simulink library "Saturation_Value_Water"  (Simulink 8.2)
settings: Solver=ode45  StartTime=0.0  StopTime=10.0  RelTol=1e-3
undefined symbols (not defined in the file): CarnotCallbacks_Saturation_Value_Water
settings Model: Creator=lena.frank  LastModifiedBy=drhf

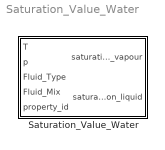
== system Saturation_Value_Water ==
  Saturation_Value_Water : Subsystem  LoadFcn=CarnotCallbacks_Saturation_Value_Water('LoadFcn');  InitFcn=load('THB.mat');  VariantControl=CarlibClassic  mask(saturation value water){INPUTARGUMENTS=state variables (classic), DEBUGLEVEL=WARNINGLEVEL, MAXTOTALMESSAGES=inf, MAXCONSECUTIVEMESSAGES=inf, WRITETOFILE=0, FILENAME='errors.txt'}
      mask prompts: INPUTARGUMENTS "Input arguments"; DEBUGLEVEL "Debug level"; MAXTOTALMESSAGES "maximum number of total warning"; MAXCONSECUTIVEMESSAGES "maximum number of consecutive warnings"; WRITETOFILE "write messages to file"; FILENAME "filename for error messages"
      mask help:
      | Calculates the saturation value of fluid by the value of a specified property.
      | Temperature may be a scalar or vector, all other inputs must be scalar.
      | property-ID        property                       unit
      | 1                       density                         [kg/m³]
      | 2                       heat capacity               [J/kgK]
      | 3                       heat conductivity         [W/mK]
      | 4                       kinematic viscosity       [m²/s]
      | 5                       enthalpy                       [J/kg]
      | 6                       entropy                         [J/kgK]
      | 7                       prandtl                          [-]
      | 8                       specific volume            [m³/kg]
      | not defined for this function
      | 9                       evaporation  enthalpy  [J/kg]
      | 10                     vapourpressure            [Pa]
      | 11                     saturationtemperatur    [°C]
      mask init:
      | %Inports
      | CarnotCallbacks_Saturation_Value_Water('CreateInports');
      | 
      | %global debug level
      | [DEBUGLEVEL, MAXTOTALMESSAGES, MAXCONSECUTIVEMESSAGES, WRITETOFILE, FILENAME] = CarnotCallbacks_Saturation_Value_Water('CheckDebugLevels', DEBUGLEVEL, MAXTOTALMESSAGES, MAXCONSECUTIVEMESSAGES, WRITETOFILE, FILENAME);
      mask Help: web(fullfile(path_carnot('help'),'saturationvalue_water.html'),'-helpbrowser')
      mask TypeOptions INPUTARGUMENTS: state variables (classic) | THB | THV
      mask Callback INPUTARGUMENTS: CarnotCallbacks_Saturation_Value_Water('MaskVisibilities');
      mask TypeOptions DEBUGLEVEL: DEBUGLEVEL | INFOLEVEL | WARNINGLEVEL | ERRORLEVEL | FATALLEVEL | NOLEVEL

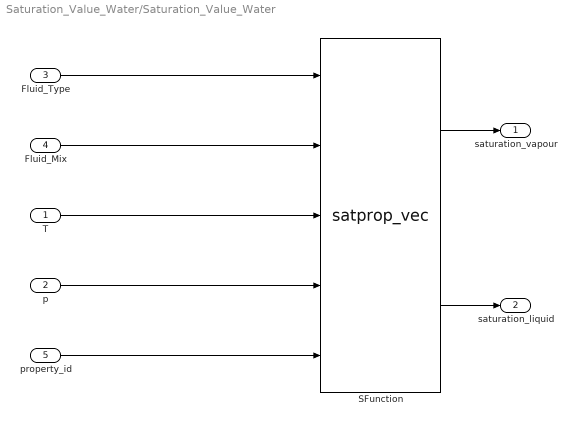
== system Saturation_Value_Water/Saturation_Value_Water ==
  T : Inport
  p : Inport  Port=2
  Fluid_Type : Inport  Port=3
  Fluid_Mix : Inport  Port=4
  property_id : Inport  Port=5
  SFunction : S-Function  FunctionName=satprop_vec  Parameters=DEBUGLEVEL,MAXTOTALMESSAGES,MAXCONSECUTIVEMESSAGES,WRITETOFILE,FILENAME  EnableBusSupport=off
  saturation_vapour : Outport
  saturation_liquid : Outport  Port=2
  wires:
  SFunction/2 -> saturation_liquid/1
  SFunction/1 -> saturation_vapour/1
  T/1 -> SFunction/3
  p/1 -> SFunction/4
  Fluid_Type/1 -> SFunction/1
  Fluid_Mix/1 -> SFunction/2
  property_id/1 -> SFunction/5
